simulink model "modelsim"  (R2025a)
settings: Solver=ode23t  StartTime=0.0  StopTime=10.0  MaxStep=0.01  RelTol=1e-3
undefined symbols (not defined in the file or in its folder): X, Y, Z
libraries: sm_lib x91, nesl_utility x20, slpidlib x1
(part 1 of 3)
settings Model: Creator=CosmosMount  LastModifiedBy=CosmosMount
settings HardwareCC: ProdHWDeviceType=AMD->x86-64 (Windows64)

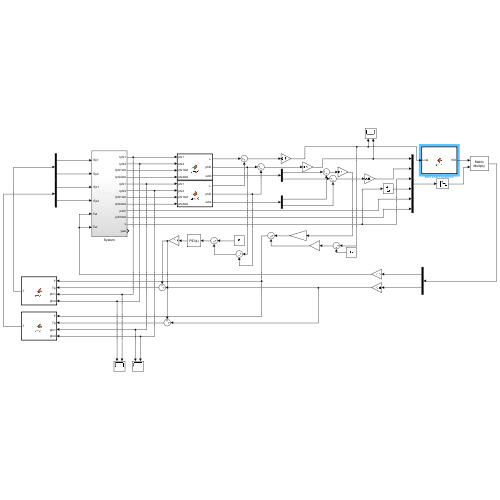
[thumbnail: Simulink's stored preview of the top-level diagram]
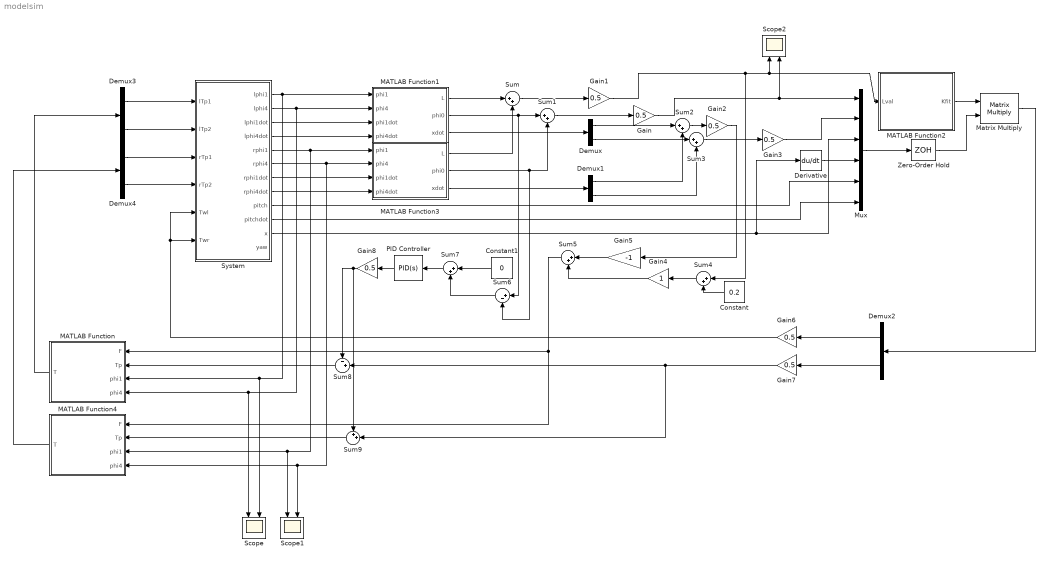
== system modelsim ==
  Constant : Constant  Value=0.2
  Constant1 : Constant  Value=0
  Demux{,1..4} (5 alike) : Demux  Outputs=2
  Derivative : Derivative
  Gain{,1..3,6..8} (7 alike) : Gain  Gain=0.5
  Gain4 : Gain
  Gain5 : Gain  Gain=-1
  MATLAB Function : MATLAB Function  TreatAsAtomicUnit=on
  MATLAB Function1 : MATLAB Function  TreatAsAtomicUnit=on
  MATLAB Function2 : MATLAB Function  TreatAsAtomicUnit=on
  MATLAB Function3 : MATLAB Function  TreatAsAtomicUnit=on
  MATLAB Function4 : MATLAB Function  TreatAsAtomicUnit=on
  Matrix Multiply : Product  Multiplication=Matrix(*)
  Mux : Mux  Inputs=6
  PID Controller : slpidlib/PID Controller  Controller=PID  Form=Parallel  TimeDomain=Continuous-time  UseExternalTs=off  SampleTime=-1  IntegratorMethod=Forward Euler  FilterMethod=Forward Euler  ControllerParametersSource=internal  P=1  I=1  UseKiTs=off  D=0  UseExternalDerivativeSource=off  N=100  UseFilter=on  TunerSelectOption=Transfer Function Based (PID Tuner App)  InitialConditionSource=internal  InitialConditionForIntegrator=0  InitialConditionForFilter=0  DifferentiatorICPrevScaledInput=0  ExternalReset=none  TrackingMode=off  Kt=1  LimitOutput=off  SatLimitsSource=internal  UpperSaturationLimit=inf  LowerSaturationLimit=-inf  LinearizeAsGain=on  AntiWindupMode=none  Kb=1  LimitIntegrator=off  UpperIntegratorSaturationLimit=inf  LowerIntegratorSaturationLimit=-inf  POutMin=[]  POutMax=[]  IOutMin=[]  IOutMax=[]  DOutMin=[]  DOutMax=[]  NOutMin=[]  NOutMax=[]  SumOutMin=[]  SumOutMax=[]  SaturationOutMin=[]  SaturationOutMax=[]  PParamMin=[]  PParamMax=[]  IParamMin=[]  IParamMax=[]  DParamMin=[]  DParamMax=[]  NParamMin=[]  NParamMax=[]  KbParamMin=[]  KbParamMax=[]  KtParamMin=[]  KtParamMax=[]  KbOutMin=[]  KbOutMax=[]  KtOutMin=[]  KtOutMax=[]  IntegratorOutMin=[]  IntegratorOutMax=[]  FilterOutMin=[]  FilterOutMax=[]  SumI1OutMin=[]  SumI1OutMax=[]  SumI2OutMin=[]  SumI2OutMax=[]  SumI3OutMin=[]  SumI3OutMax=[]  SumI4OutMin=[]  SumI4OutMax=[]  SumDOutMin=[]  SumDOutMax=[]  DifferentiatorOutMin=[]  DifferentiatorOutMax=[]  FilterDiffOutCoefMin=[]  FilterDiffOutCoefMax=[]  ReciprocalOutMin=[]  ReciprocalOutMax=[]  SumDenOutMin=[]  SumDenOutMax=[]  SumNumOutMin=[]  SumNumOutMax=[]  DivideOutMin=[]  DivideOutMax=[]  UdiffTsProdOutMin=[]  UdiffTsProdOutMax=[]  NTsProdOutMin=[]  NTsProdOutMax=[]  UintegralTsProdOutMin=[]  UintegralTsProdOutMax=[]  UngainTsProdOutMin=[]  UngainTsProdOutMax=[]  ClampingZeroOutDataTypeStr=Inherit: Inherit via back propagation  ClampingZeroOutMin=[]  ClampingZeroOutMax=[]  FilterDenConstantOutDataTypeStr=Inherit: Inherit via back propagation  FilterDenConstantOutMin=[]  FilterDenConstantOutMax=[]  PCopyOutDataTypeStr=Inherit: Inherit via back propagation  PCopyOutMin=[]  PCopyOutMax=[]  NCopyOutDataTypeStr=Inherit: Inherit via back propagation  NCopyOutMin=[]  NCopyOutMax=[]  IntegratorContinuousStateAttributes=''  IntegratorStateMustResolveToSignalObject=off  IntegratorRTWStateStorageClass=Auto  FilterContinuousStateAttributes=''  FilterStateMustResolveToSignalObject=off  FilterRTWStateStorageClass=Auto  ParallelPVariant=InternalParameters  IdealPVariant=Disabled  IVariant=InternalParameters  DVariant=InternalParameters  IntegratorVariant=Continuous  SatVariant=Disabled  AWVariant=Passthrough  PCopyVariant=Disabled  TRVariant=Disabled  FdbkBlocksVariant=Forward  IdealPFdbkVariant=Disabled  SatFdbkVariant=Disabled  DerivativeFilterVariant=ContFilter  NVariant=InternalParameters  NCopyVariant=Disabled  FilterICVariant=InternalICsFilter  IntegratorICVariant=InternalICs  ExternalResetVariant=Disabled  TRSumVariant=Passthrough  SumFdbkVariant=Disabled  SumVariant=Sum_PID  TsampFilterVariant=InternalTs  TsampNgainVariant=Passthrough  TsampIntegralVariant=Disabled_SignalSpec  ExternalSaturationOutDataTypeStr=Inherit: Same as second input  DerivativeSourceVariant=ErrorSignal  PreIntVariant=InternalPreInt
  Scope : Scope  NumInputPorts=2
  Scope1 : Scope  NumInputPorts=2
  Scope2 : Scope  NumInputPorts=2
      settings: ActiveDisplayYMinimum=-0.39172313156802929  ActiveDisplayYMaximum=0.781178459798323  DataLoggingVariableName=ScopeData2
  Sum{,1..5,7} (7 alike) : Sum  Inputs=|++
  Sum6 : Sum  Inputs=|+-
  Sum8 : Sum  Inputs=-+|
  Sum9 : Sum  Inputs=++|
  System : Subsystem
  Zero-Order Hold : ZeroOrderHold  SampleTime=0.005
  wires:
  System/1(lphi1) -> MATLAB Function1/1(phi1), MATLAB Function/3(phi1), Scope/2
  System/2(lphi4) -> MATLAB Function1/2(phi4), Scope/1, MATLAB Function/4(phi4)
  System/3(lphi1dot) -> MATLAB Function1/3(phi1dot)
  System/4(lphi4dot) -> MATLAB Function1/4(phi4dot)
  System/5(rphi1) -> MATLAB Function3/1(phi1), Scope1/1, MATLAB Function4/3(phi1)
  System/6(rphi4) -> MATLAB Function3/2(phi4), Scope1/2, MATLAB Function4/4(phi4)
  System/7(rphi1dot) -> MATLAB Function3/3(phi1dot)
  System/8(rphi4dot) -> MATLAB Function3/4(phi4dot)
  MATLAB Function1/1(L) -> Sum/1
  MATLAB Function3/1(L) -> Sum/2
  MATLAB Function1/2(phi0) -> Sum6/1, Sum1/1
  MATLAB Function3/2(phi0) -> Sum6/2, Sum1/2
  MATLAB Function1/3(xdot) -> Demux/1
  MATLAB Function3/3(xdot) -> Demux1/1
  Sum1/1 -> Gain/1
  Sum/1 -> Gain1/1
  Sum2/1 -> Gain2/1
  Demux/1 -> Sum2/1
  Demux1/1 -> Sum2/2
  Sum3/1 -> Gain3/1
  Demux/2 -> Sum3/1
  Demux1/2 -> Sum3/2
  Gain/1 -> Scope2/2, Mux/1
  Gain3/1 -> Mux/2
  System/9(pitch) -> Mux/5
  System/10(pitchdot) -> Mux/6
  System/11(x) -> Derivative/1, Mux/3
  Derivative/1 -> Mux/4
  Gain1/1 -> Sum4/1, MATLAB Function2/1(Lval), Scope2/1
  Gain2/1 -> Gain5/1
  MATLAB Function2/1(Kfit) -> Matrix Multiply/1
  Mux/1 -> Zero-Order Hold/1
  Zero-Order Hold/1 -> Matrix Multiply/2
  Matrix Multiply/1 -> Demux2/1
  Constant/1 -> Sum4/2
  Sum4/1 -> Gain4/1
  Gain5/1 -> Sum5/1
  Gain4/1 -> Sum5/2
  Sum5/1 -> MATLAB Function/1(F), MATLAB Function4/1(F)
  Constant1/1 -> Sum7/1
  Sum6/1 -> Sum7/2
  Sum7/1 -> PID Controller/1
  Demux2/1 -> Gain6/1
  Gain6/1 -> System/6(Twr), System/5(Twl)
  PID Controller/1 -> Gain8/1
  Sum8/1 -> MATLAB Function/2(Tp)
  Demux3/1 -> System/1(lTp1)
  Demux3/2 -> System/2(lTp2)
  Demux4/1 -> System/3(rTp1)
  Demux4/2 -> System/4(rTp2)
  MATLAB Function/1(T) -> Demux3/1
  MATLAB Function4/1(T) -> Demux4/1
  Demux2/2 -> Gain7/1
  Gain7/1 -> Sum9/2, Sum8/2
  Sum9/1 -> MATLAB Function4/2(Tp)
  Gain8/1 -> Sum8/1, Sum9/1
